simulink model "RoboSoccerSim"  (R2022b)
settings: Solver=ode4  StartTime=0.0  StopTime=inf  FixedStep=0.01  RelTol=1e-3
libraries: dspindex x20
(part 1 of 2)
settings Model: Creator=Wikian  LastModifiedBy=Sahil Gaurkar
settings ModelReferenceCC: EnableRefExpFcnMdlSchedulingChecks=on

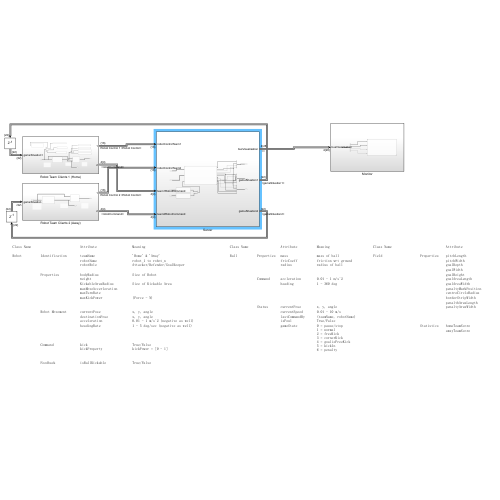
[thumbnail: Simulink's stored preview of the top-level diagram]
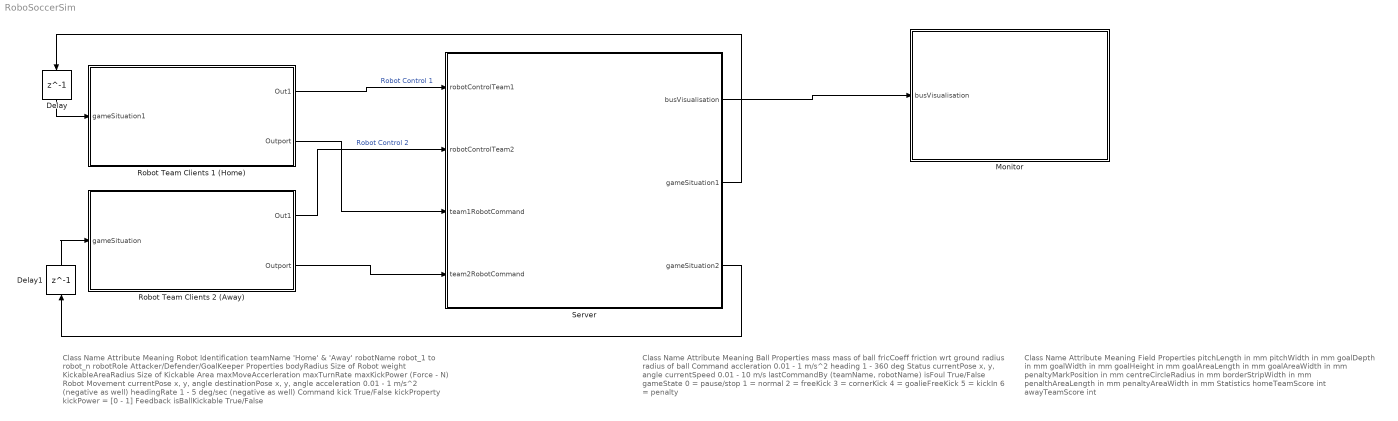
== system RoboSoccerSim ==
  note: Class Name
      |
      | Attribute
      | Meaning
      |
      | Field
      | Properties
      | pitchLength
      | in mm
      |
      | pitchWidth
      | in mm
      |
      | goalDepth
      | in mm
      |
      | goalWidth
      | in mm
      |
      | goalHeight
      | in mm
      |
      | goalAreaLength
      | in mm
      |
      | goalAreaWidth
      | in mm
      |
      | penaltyMarkPosition
      | in mm
      |
      | centreCircleRadius
      | in mm
      |
      | borderStripWidth
      | in mm
      |
      | penalthAreaLength
      | in mm
      |
      | penaltyAreaWidth
      | in mm
      |
      | Statistics
      | homeTeamScore
      | int
      |
      | awayTeamScore
      | int
  note: Class Name
      |
      | Attribute
      | Meaning
      |
      | Ball
      | Properties
      | mass
      | mass of ball
      |
      | fricCoeff
      | friction wrt ground
      |
      | radius
      | radius of ball
      |
      | Command
      | accleration
      | 0.01 - 1 m/s^2
      |
      | heading
      | 1 - 360 deg
      |
      | Status
      | currentPose
      | x, y, angle
      |
      | currentSpeed
      | 0.01 - 10 m/s
      |
      | lastCommandBy
      | (teamName, robotName)
      |
      | isFoul
      | True/False
      |
      | gameState
      | 0 = pause/stop
      | 1 = normal
      | 2 = freeKick
      | 3 = cornerKick
      | 4 = goalieFreeKick
      | 5 = kickIn
      | 6 = penalty
  note: Class Name
      |
      | Attribute
      | Meaning
      |
      | Robot
      | Identification
      | teamName
      | 'Home' & 'Away'
      |
      | robotName
      | robot_1 to robot_n
      |
      | robotRole
      | Attacker/Defender/GoalKeeper
      |
      | Properties
      | bodyRadius
      | Size of Robot
      |
      | weight
      |
      | KickableAreaRadius
      | Size of Kickable Area
      |
      | maxMoveAccerleration
      |
      | maxTurnRate
      |
      | maxKickPower
      | (Force - N)
      |
      | Robot Movement
      | currentPose
      | x, y, angle
      |
      | destinationPose
      | x, y, angle
      |
      | acceleration
      | 0.01 - 1 m/s^2 (negative as well)
      |
      | headingRate
      | 1 - 5 deg/sec (negative as well)
      |
      | Command
      | kick
      | True/False
      |
      | kickProperty
      | kickPower = [0 - 1]
      |
      | Feedback
      | isBallKickable
      | True/False
  Delay : Delay  DelayLength=1
  Delay1 : Delay  DelayLength=1
  Monitor : Subsystem
  Robot Team Clients 1 (Home) : Subsystem
  Robot Team Clients 2 (Away) : Subsystem
  Server : Subsystem
  wires:
  Robot Team Clients 1 (Home)/1(Out1) -> Server/1(robotControlTeam1)  "Robot Control 1"
  Robot Team Clients 2 (Away)/1(Out1) -> Server/2(robotControlTeam2)  "Robot Control 2"
  Server/1(busVisualisation) -> Monitor/1(busVisualisation)
  Server/3(gameSituation2) -> Delay1/1
  Server/2(gameSituation1) -> Delay/1
  Delay/1 -> Robot Team Clients 1 (Home)/1(gameSituation1)
  Delay1/1 -> Robot Team Clients 2 (Away)/1(gameSituation)
  Robot Team Clients 1 (Home)/2(Outport) -> Server/3(team1RobotCommand)
  Robot Team Clients 2 (Away)/2(Outport) -> Server/4(team2RobotCommand)

== system RoboSoccerSim/Monitor ==
  busVisualisation : Inport
  Bus Selector : BusSelector  OutputSignals=robot coordinates and heading,ballCurrentPose,home team score,away team score
  Subsystem Reference : Subsystem  ReferencedSubsystem=Monitor_Subsystem
  wires:
  busVisualisation/1 -> Bus Selector/1
  Bus Selector/1 -> Subsystem Reference/1  "<robot coordinates and heading>"
  Bus Selector/2 -> Subsystem Reference/2  "<ballCurrentPose>"
  Bus Selector/3 -> Subsystem Reference/3  "<home team score>"
  Bus Selector/4 -> Subsystem Reference/4  "<away team score>"

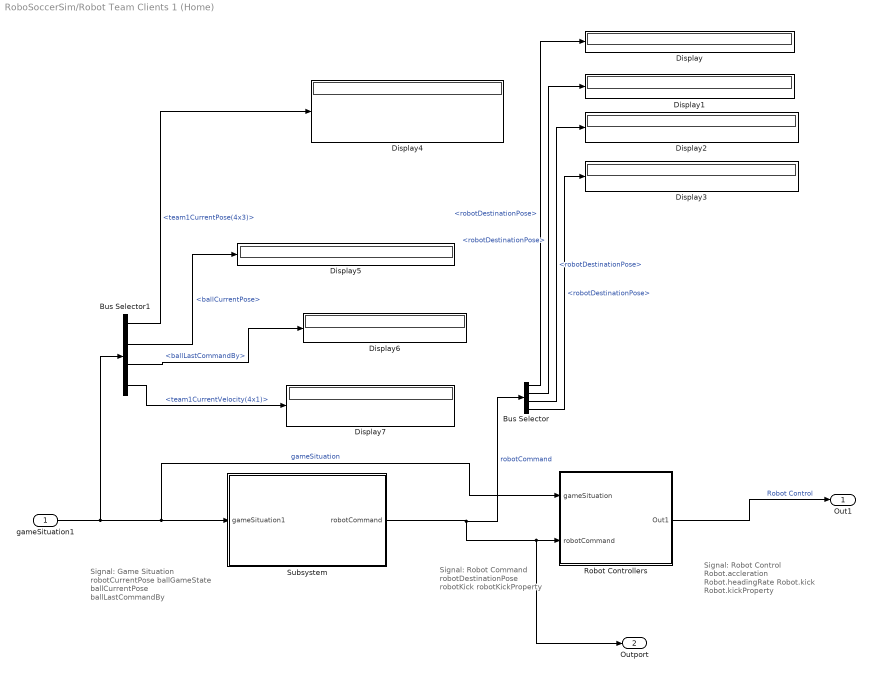
== system RoboSoccerSim/Robot Team Clients 1 (Home) ==
  note: Signal: Robot Control
      |
      | 	Robot.accleration
      | 	Robot.headingRate
      | 	Robot.kick
      | 	Robot.kickProperty
  note: Signal: Robot Command
      |
      | 	robotDestinationPose
      | 	robotKick
      | 	robotKickProperty
  note: Signal: Game Situation
      | 	robotCurrentPose
      | 	ballGameState
      | 	ballCurrentPose
      | 	ballLastCommandBy
  gameSituation1 : Inport  OutDataTypeStr=Bus: gameSituation
  Bus Selector : BusSelector  OutputSignals=robot1.robotDestinationPose,robot2.robotDestinationPose,robot3.robotDestinationPose,robot4.robotDestinationPose
  Bus Selector1 : BusSelector  OutputSignals=team1CurrentPose(4x3),ballCurrentPose,ballLastCommandBy,team1CurrentVelocity(4x1)
  Display{,1..7} (8 alike) : Display
  Robot Controllers : Subsystem
  Subsystem : Subsystem
  Out1 : Outport
  Outport : Outport  Port=2
  wires:
  gameSituation1/1 -> Bus Selector1/1, Subsystem/1(gameSituation1), Robot Controllers/1(gameSituation)  "gameSituation"
  Subsystem/1(robotCommand) -> Bus Selector/1, Outport/1, Robot Controllers/2(robotCommand)  "robotCommand"
  Robot Controllers/1(Out1) -> Out1/1  "Robot Control"
  Bus Selector/1 -> Display/1  "<robotDestinationPose>"
  Bus Selector/2 -> Display1/1  "<robotDestinationPose>"
  Bus Selector/3 -> Display2/1  "<robotDestinationPose>"
  Bus Selector/4 -> Display3/1  "<robotDestinationPose>"
  Bus Selector1/1 -> Display4/1  "<team1CurrentPose(4x3)>"
  Bus Selector1/2 -> Display5/1  "<ballCurrentPose>"
  Bus Selector1/3 -> Display6/1  "<ballLastCommandBy>"
  Bus Selector1/4 -> Display7/1  "<team1CurrentVelocity(4x1)>"

== system RoboSoccerSim/Robot Team Clients 2 (Away) ==
  note: Signal: Robot Control
      |
      | 	Robot.accleration
      | 	Robot.headingRate
      | 	Robot.kick
      | 	Robot.kickProperty
  note: Signal: Robot Command
      |
      | 	robotDestinationPose
      | 	robotKick
      | 	robotKickProperty
  note: Signal: Game Situation
      | 	robotCurrentPose
      | 	ballGameState
      | 	ballCurrentPose
      | 	ballLastCommandBy
  gameSituation : Inport  OutDataTypeStr=Bus:gameSituation
  Robot Controllers : Subsystem
  Subsystem : Subsystem
  Out1 : Outport
  Outport : Outport  Port=2
  wires:
  gameSituation/1 -> Subsystem/1(gameSituation1), Robot Controllers/1(gameSituation)  "gameSituation"
  Subsystem/1(robotCommand) -> Outport/1, Robot Controllers/2(robotCommand)  "robotCommand"
  Robot Controllers/1(Out1) -> Out1/1  "Robot Control"

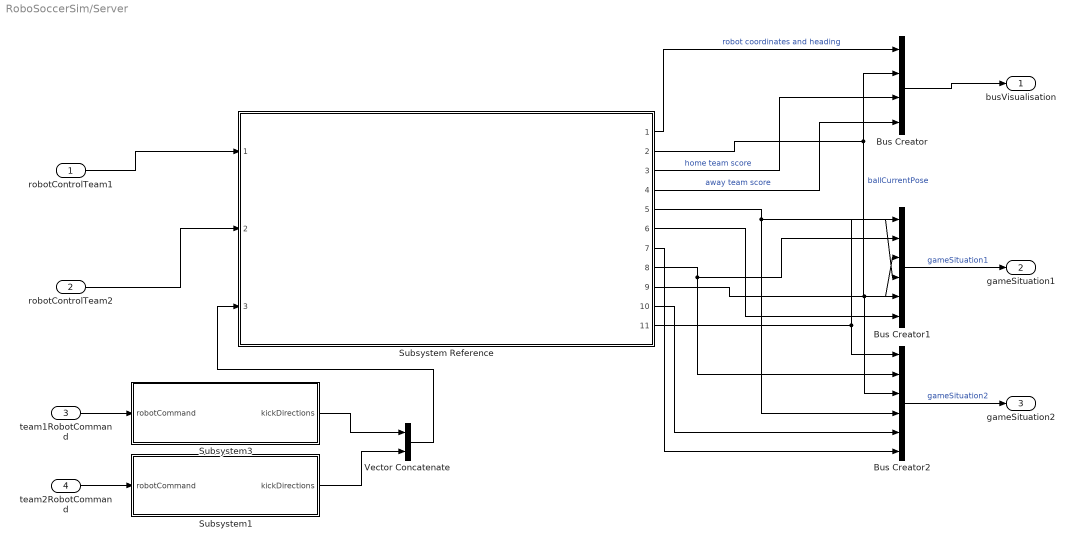
== system RoboSoccerSim/Server ==
  robotControlTeam1 : Inport
  robotControlTeam2 : Inport  Port=2
  team1RobotCommand : Inport  Port=3
  team2RobotCommand : Inport  Port=4
  Bus Creator : BusCreator  Inputs=4
  Bus Creator1 : BusCreator  Inputs=6  OutDataTypeStr=Bus: gameSituation
  Bus Creator2 : BusCreator  Inputs=6  OutDataTypeStr=Bus: gameSituation
  Subsystem Reference : Subsystem  ReferencedSubsystem=Server_sub
  Subsystem1 : Subsystem
  Subsystem3 : Subsystem
  Vector Concatenate : Concatenate
  busVisualisation : Outport
  gameSituation1 : Outport  Port=2
  gameSituation2 : Outport  Port=3
  wires:
  robotControlTeam2/1 -> Subsystem Reference/2
  robotControlTeam1/1 -> Subsystem Reference/1
  Subsystem Reference/1 -> Bus Creator/1  "robot coordinates and heading"
  Subsystem Reference/2 -> Bus Creator/2, Bus Creator2/3, Bus Creator1/3  "ballCurrentPose"
  Subsystem Reference/3 -> Bus Creator/3  "home team score"
  Subsystem Reference/4 -> Bus Creator/4  "away team score"
  Subsystem Reference/5 -> Bus Creator2/4, Bus Creator1/4
  Bus Creator/1 -> busVisualisation/1
  Subsystem Reference/6 -> Bus Creator1/6
  Subsystem Reference/8 -> Bus Creator2/2, Bus Creator1/2
  Subsystem Reference/9 -> Bus Creator1/5
  Subsystem Reference/11 -> Bus Creator2/1, Bus Creator1/1
  Bus Creator1/1 -> gameSituation1/1  "gameSituation1"
  Subsystem Reference/7 -> Bus Creator2/6
  Subsystem Reference/10 -> Bus Creator2/5
  Bus Creator2/1 -> gameSituation2/1  "gameSituation2"
  Vector Concatenate/1 -> Subsystem Reference/3
  team2RobotCommand/1 -> Subsystem1/1(robotCommand)
  Subsystem1/1(kickDirections) -> Vector Concatenate/2
  team1RobotCommand/1 -> Subsystem3/1(robotCommand)
  Subsystem3/1(kickDirections) -> Vector Concatenate/1

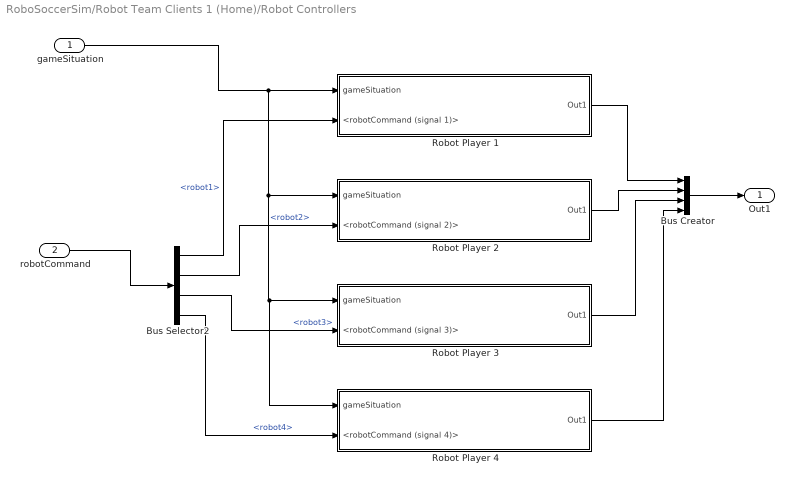
== system RoboSoccerSim/Robot Team Clients 1 (Home)/Robot Controllers ==
  gameSituation : Inport
  robotCommand : Inport  Port=2
  Bus Creator : BusCreator  Inputs=4
  Bus Selector2 : BusSelector  OutputSignals=robot1,robot2,robot3,robot4
  Robot Player 1 : Subsystem
  Robot Player 2 : Subsystem
  Robot Player 3 : Subsystem
  Robot Player 4 : Subsystem
  Out1 : Outport
  wires:
  Robot Player 1/1(Out1) -> Bus Creator/1
  Bus Creator/1 -> Out1/1
  robotCommand/1 -> Bus Selector2/1
  Bus Selector2/1 -> Robot Player 1/2(<robotCommand (signal 1)>)  "<robot1>"
  gameSituation/1 -> Robot Player 4/1(gameSituation), Robot Player 3/1(gameSituation), Robot Player 2/1(gameSituation), Robot Player 1/1(gameSituation)
  Bus Selector2/2 -> Robot Player 2/2(<robotCommand (signal 2)>)  "<robot2>"
  Bus Selector2/3 -> Robot Player 3/2(<robotCommand (signal 3)>)  "<robot3>"
  Robot Player 2/1(Out1) -> Bus Creator/2
  Robot Player 3/1(Out1) -> Bus Creator/3
  Robot Player 4/1(Out1) -> Bus Creator/4
  Bus Selector2/4 -> Robot Player 4/2(<robotCommand (signal 4)>)  "<robot4>"

== system RoboSoccerSim/Robot Team Clients 1 (Home)/Subsystem ==
  gameSituation1 : Inport  OutDataTypeStr=Bus: gameSituation
  Bus Creator : BusCreator  Inputs=4
  Bus Selector : BusSelector  OutputSignals=robotDestinationPose
  Display : Display
  Home Player Strategy 1 : Stateflow chart  TreatAsAtomicUnit=on
  Home Player Strategy 2 : Stateflow chart  TreatAsAtomicUnit=on
  Home Player Strategy 3 : Stateflow chart  TreatAsAtomicUnit=on
  Home Player Strategy 4 : Stateflow chart  TreatAsAtomicUnit=on
  robotCommand : Outport
  wires:
  Home Player Strategy 3/1(robotCommand) -> Bus Creator/3  "robot3"
  gameSituation1/1 -> Home Player Strategy 2/1(gameSituation), Home Player Strategy 1/1(gameSituation), Home Player Strategy 4/1(gameSituation), Home Player Strategy 3/1(gameSituation)  "gameSituation1"
  Home Player Strategy 2/1(robotCommand) -> Bus Creator/2  "robot2"
  Bus Selector/1 -> Display/1  "<robotDestinationPose>"
  Home Player Strategy 4/1(robotCommand) -> Bus Creator/4  "robot4"
  Home Player Strategy 1/1(robotCommand) -> Bus Selector/1, Bus Creator/1  "robot1"
  Bus Creator/1 -> robotCommand/1

== system RoboSoccerSim/Robot Team Clients 2 (Away)/Robot Controllers ==
  gameSituation : Inport
  robotCommand : Inport  Port=2
  Bus Creator : BusCreator  Inputs=4
  Bus Selector2 : BusSelector  OutputSignals=robot1,robot2,robot3,robot4
  Robot Player 1 : Subsystem
  Robot Player 2 : Subsystem
  Robot Player 3 : Subsystem
  Robot Player 4 : Subsystem
  Out1 : Outport
  wires:
  Robot Player 1/1(Out1) -> Bus Creator/1
  Bus Creator/1 -> Out1/1
  robotCommand/1 -> Bus Selector2/1
  Bus Selector2/1 -> Robot Player 1/2(<robotCommand (signal 1)>)  "<robot1>"
  gameSituation/1 -> Robot Player 4/1(gameSituation), Robot Player 3/1(gameSituation), Robot Player 2/1(gameSituation), Robot Player 1/1(gameSituation)
  Bus Selector2/2 -> Robot Player 2/2(<robotCommand (signal 2)>)  "<robot2>"
  Bus Selector2/3 -> Robot Player 3/2(<robotCommand (signal 3)>)  "<robot3>"
  Robot Player 2/1(Out1) -> Bus Creator/2
  Robot Player 3/1(Out1) -> Bus Creator/3
  Robot Player 4/1(Out1) -> Bus Creator/4
  Bus Selector2/4 -> Robot Player 4/2(<robotCommand (signal 4)>)  "<robot4>"

== system RoboSoccerSim/Robot Team Clients 2 (Away)/Subsystem ==
  gameSituation1 : Inport  OutDataTypeStr=Bus: gameSituation
  Away Player Strategy 1 : Stateflow chart  TreatAsAtomicUnit=on
  Away Player Strategy 2 : Stateflow chart  TreatAsAtomicUnit=on
  Away Player Strategy 3 : Stateflow chart  TreatAsAtomicUnit=on
  Away Player Strategy 4 : Stateflow chart  TreatAsAtomicUnit=on
  Bus Creator : BusCreator  Inputs=4
  Bus Selector : BusSelector  OutputSignals=robotDestinationPose
  Display : Display
  robotCommand : Outport
  wires:
  Away Player Strategy 3/1(robotCommand) -> Bus Creator/3  "robot3"
  gameSituation1/1 -> Away Player Strategy 2/1(gameSituation), Away Player Strategy 1/1(gameSituation), Away Player Strategy 4/1(gameSituation), Away Player Strategy 3/1(gameSituation)  "gameSituation1"
  Away Player Strategy 2/1(robotCommand) -> Bus Creator/2  "robot2"
  Bus Selector/1 -> Display/1  "<robotDestinationPose>"
  Away Player Strategy 4/1(robotCommand) -> Bus Creator/4  "robot4"
  Away Player Strategy 1/1(robotCommand) -> Bus Creator/1, Bus Selector/1  "robot1"
  Bus Creator/1 -> robotCommand/1

== system RoboSoccerSim/Server/Subsystem1 ==
  note: Signal: Robot Control
      |
      | 	Robot.accleration
      | 	Robot.headingRate
      | 	Robot.kick
      | 	Robot.kickProperty
  robotCommand : Inport
  Bus Selector2 : BusSelector  OutputSignals=robot1.robotDestinationPose,robot2.robotDestinationPose,robot3.robotDestinationPose,robot4.robotDestinationPose
  MATLAB Function : MATLAB Function  TreatAsAtomicUnit=on
  MATLAB Function1 : MATLAB Function  TreatAsAtomicUnit=on
  MATLAB Function2 : MATLAB Function  TreatAsAtomicUnit=on
  MATLAB Function3 : MATLAB Function  TreatAsAtomicUnit=on
  Vector Concatenate : Concatenate  NumInputs=4
  kickDirections : Outport
  wires:
  MATLAB Function/1(kickDirection) -> Vector Concatenate/1
  Vector Concatenate/1 -> kickDirections/1
  MATLAB Function1/1(kickDirection) -> Vector Concatenate/2
  robotCommand/1 -> Bus Selector2/1
  Bus Selector2/4 -> MATLAB Function3/1(destinationPose)  "<robotDestinationPose>"
  Bus Selector2/1 -> MATLAB Function/1(destinationPose)  "<robotDestinationPose>"
  MATLAB Function2/1(kickDirection) -> Vector Concatenate/3
  Bus Selector2/2 -> MATLAB Function1/1(destinationPose)  "<robotDestinationPose>"
  Bus Selector2/3 -> MATLAB Function2/1(destinationPose)  "<robotDestinationPose>"
  MATLAB Function3/1(kickDirection) -> Vector Concatenate/4

== system RoboSoccerSim/Server/Subsystem3 ==
  note: Signal: Robot Control
      |
      | 	Robot.accleration
      | 	Robot.headingRate
      | 	Robot.kick
      | 	Robot.kickProperty
  robotCommand : Inport
  Bus Selector2 : BusSelector  OutputSignals=robot1.robotDestinationPose,robot2.robotDestinationPose,robot3.robotDestinationPose,robot4.robotDestinationPose
  MATLAB Function : MATLAB Function  TreatAsAtomicUnit=on
  MATLAB Function1 : MATLAB Function  TreatAsAtomicUnit=on
  MATLAB Function2 : MATLAB Function  TreatAsAtomicUnit=on
  MATLAB Function3 : MATLAB Function  TreatAsAtomicUnit=on
  Vector Concatenate : Concatenate  NumInputs=4
  kickDirections : Outport
  wires:
  MATLAB Function/1(kickDirection) -> Vector Concatenate/1
  Vector Concatenate/1 -> kickDirections/1
  MATLAB Function1/1(kickDirection) -> Vector Concatenate/2
  robotCommand/1 -> Bus Selector2/1
  Bus Selector2/4 -> MATLAB Function3/1(destinationPose)  "<robotDestinationPose>"
  Bus Selector2/1 -> MATLAB Function/1(destinationPose)  "<robotDestinationPose>"
  MATLAB Function2/1(kickDirection) -> Vector Concatenate/3
  Bus Selector2/2 -> MATLAB Function1/1(destinationPose)  "<robotDestinationPose>"
  Bus Selector2/3 -> MATLAB Function2/1(destinationPose)  "<robotDestinationPose>"
  MATLAB Function3/1(kickDirection) -> Vector Concatenate/4

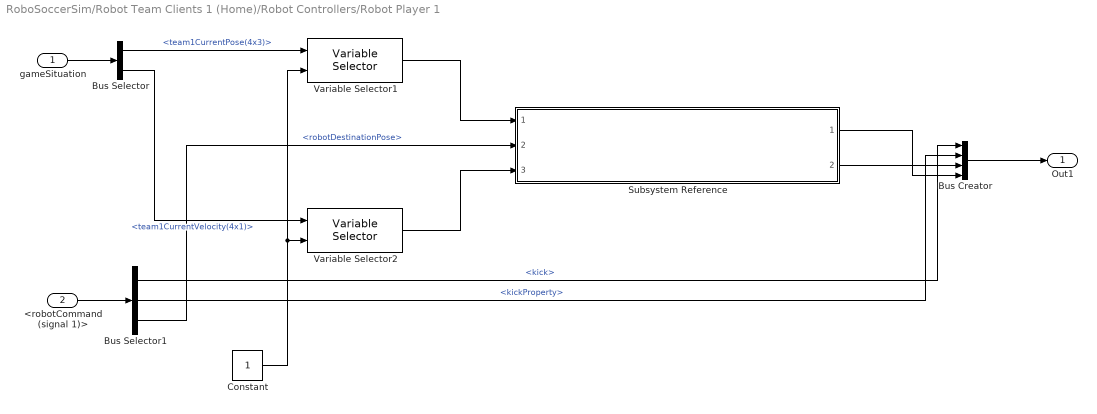
== system RoboSoccerSim/Robot Team Clients 1 (Home)/Robot Controllers/Robot Player 1 ==
  gameSituation : Inport
  <robotCommand (signal 1)> : Inport  Port=2
  Bus Creator : BusCreator  Inputs=4  OutDataTypeStr=Bus: robotControl
  Bus Selector : BusSelector  OutputSignals=team1CurrentPose(4x3),team1CurrentVelocity(4x1)
  Bus Selector1 : BusSelector  OutputSignals=kick,kickProperty,robotDestinationPose
  Constant : Constant
  Subsystem Reference : Subsystem  ReferencedSubsystem=Controller_Subsystem
  Variable Selector1 : dspindex/Variable Selector  NumInputs=1  rowsOrCols=Rows  IdxMode=Variable  Elements=[1 3]  ZerOneIdxMode=One-based  errmode=Clip Index  FillMode=on  FillValues=0
      settings: LibrarySourceBlock=|
      | dsphdlsupportsigmgmt/Variable
      | Selector
  Variable Selector2 : dspindex/Variable Selector  NumInputs=1  rowsOrCols=Rows  IdxMode=Variable  Elements=[1 3]  ZerOneIdxMode=One-based  errmode=Clip Index  FillMode=on  FillValues=0
      settings: LibrarySourceBlock=|
      | dsphdlsupportsigmgmt/Variable
      | Selector
  Out1 : Outport
  wires:
  Bus Selector1/3 -> Subsystem Reference/2  "<robotDestinationPose>"
  Constant/1 -> Variable Selector2/2, Variable Selector1/2
  Variable Selector1/1 -> Subsystem Reference/1
  Variable Selector2/1 -> Subsystem Reference/3
  gameSituation/1 -> Bus Selector/1
  Bus Selector/1 -> Variable Selector1/1  "<team1CurrentPose(4x3)>"
  Bus Selector/2 -> Variable Selector2/1  "<team1CurrentVelocity(4x1)>"
  <robotCommand (signal 1)>/1 -> Bus Selector1/1
  Bus Selector1/1 -> Bus Creator/1  "<kick>"
  Bus Selector1/2 -> Bus Creator/2  "<kickProperty>"
  Subsystem Reference/1 -> Bus Creator/4
  Subsystem Reference/2 -> Bus Creator/3
  Bus Creator/1 -> Out1/1

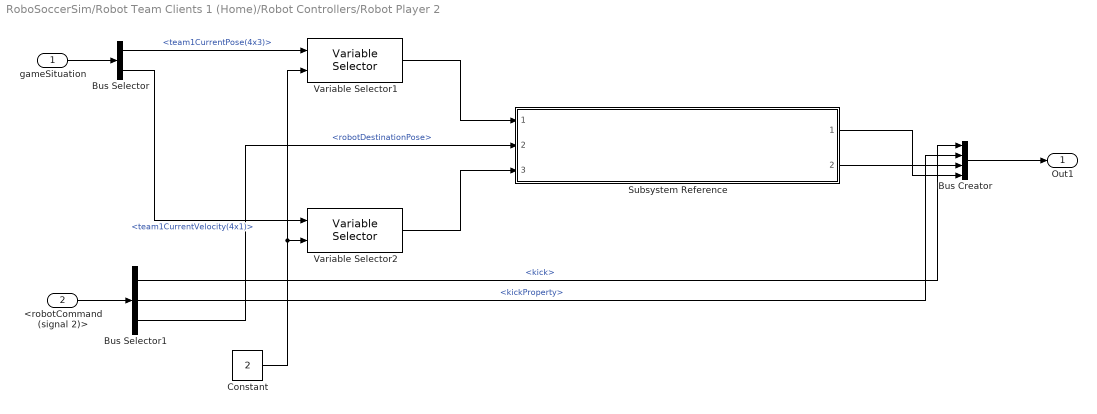
== system RoboSoccerSim/Robot Team Clients 1 (Home)/Robot Controllers/Robot Player 2 ==
  gameSituation : Inport
  <robotCommand (signal 2)> : Inport  Port=2
  Bus Creator : BusCreator  Inputs=4  OutDataTypeStr=Bus: robotControl
  Bus Selector : BusSelector  OutputSignals=team1CurrentPose(4x3),team1CurrentVelocity(4x1)
  Bus Selector1 : BusSelector  OutputSignals=kick,kickProperty,robotDestinationPose
  Constant : Constant  Value=2
  Subsystem Reference : Subsystem  ReferencedSubsystem=Controller_Subsystem
  Variable Selector1 : dspindex/Variable Selector  NumInputs=1  rowsOrCols=Rows  IdxMode=Variable  Elements=[1 3]  ZerOneIdxMode=One-based  errmode=Clip Index  FillMode=on  FillValues=0
      settings: LibrarySourceBlock=|
      | dsphdlsupportsigmgmt/Variable
      | Selector
  Variable Selector2 : dspindex/Variable Selector  NumInputs=1  rowsOrCols=Rows  IdxMode=Variable  Elements=[1 3]  ZerOneIdxMode=One-based  errmode=Clip Index  FillMode=on  FillValues=0
      settings: LibrarySourceBlock=|
      | dsphdlsupportsigmgmt/Variable
      | Selector
  Out1 : Outport
  wires:
  Constant/1 -> Variable Selector2/2, Variable Selector1/2
  Variable Selector1/1 -> Subsystem Reference/1
  Variable Selector2/1 -> Subsystem Reference/3
  gameSituation/1 -> Bus Selector/1
  Bus Selector/1 -> Variable Selector1/1  "<team1CurrentPose(4x3)>"
  Bus Selector/2 -> Variable Selector2/1  "<team1CurrentVelocity(4x1)>"
  <robotCommand (signal 2)>/1 -> Bus Selector1/1
  Bus Selector1/1 -> Bus Creator/1  "<kick>"
  Bus Selector1/2 -> Bus Creator/2  "<kickProperty>"
  Subsystem Reference/1 -> Bus Creator/4
  Subsystem Reference/2 -> Bus Creator/3
  Bus Creator/1 -> Out1/1
  Bus Selector1/3 -> Subsystem Reference/2  "<robotDestinationPose>"

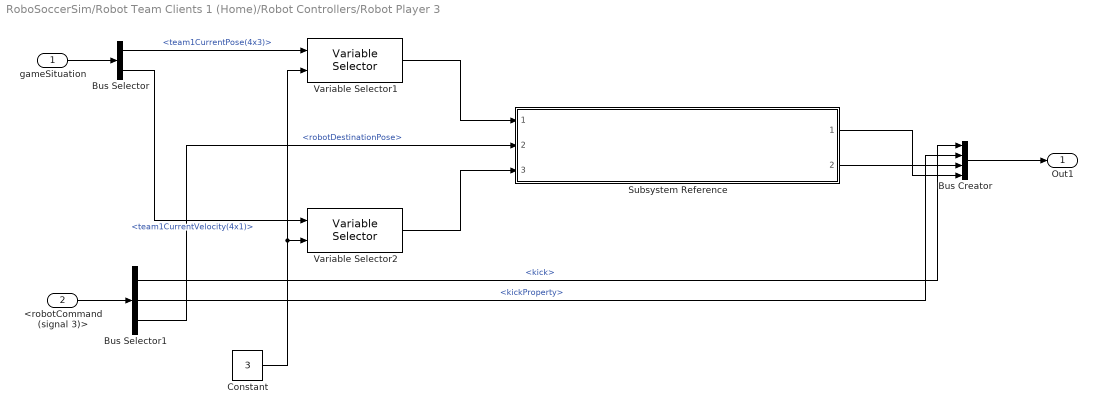
== system RoboSoccerSim/Robot Team Clients 1 (Home)/Robot Controllers/Robot Player 3 ==
  gameSituation : Inport
  <robotCommand (signal 3)> : Inport  Port=2
  Bus Creator : BusCreator  Inputs=4  OutDataTypeStr=Bus: robotControl
  Bus Selector : BusSelector  OutputSignals=team1CurrentPose(4x3),team1CurrentVelocity(4x1)
  Bus Selector1 : BusSelector  OutputSignals=kick,kickProperty,robotDestinationPose
  Constant : Constant  Value=3
  Subsystem Reference : Subsystem  ReferencedSubsystem=Controller_Subsystem
  Variable Selector1 : dspindex/Variable Selector  NumInputs=1  rowsOrCols=Rows  IdxMode=Variable  Elements=[1 3]  ZerOneIdxMode=One-based  errmode=Clip Index  FillMode=on  FillValues=0
      settings: LibrarySourceBlock=|
      | dsphdlsupportsigmgmt/Variable
      | Selector
  Variable Selector2 : dspindex/Variable Selector  NumInputs=1  rowsOrCols=Rows  IdxMode=Variable  Elements=[1 3]  ZerOneIdxMode=One-based  errmode=Clip Index  FillMode=on  FillValues=0
      settings: LibrarySourceBlock=|
      | dsphdlsupportsigmgmt/Variable
      | Selector
  Out1 : Outport
  wires:
  Bus Selector1/3 -> Subsystem Reference/2  "<robotDestinationPose>"
  Constant/1 -> Variable Selector2/2, Variable Selector1/2
  Variable Selector1/1 -> Subsystem Reference/1
  Variable Selector2/1 -> Subsystem Reference/3
  gameSituation/1 -> Bus Selector/1
  Bus Selector/1 -> Variable Selector1/1  "<team1CurrentPose(4x3)>"
  Bus Selector/2 -> Variable Selector2/1  "<team1CurrentVelocity(4x1)>"
  <robotCommand (signal 3)>/1 -> Bus Selector1/1
  Bus Selector1/1 -> Bus Creator/1  "<kick>"
  Bus Selector1/2 -> Bus Creator/2  "<kickProperty>"
  Subsystem Reference/1 -> Bus Creator/4
  Subsystem Reference/2 -> Bus Creator/3
  Bus Creator/1 -> Out1/1

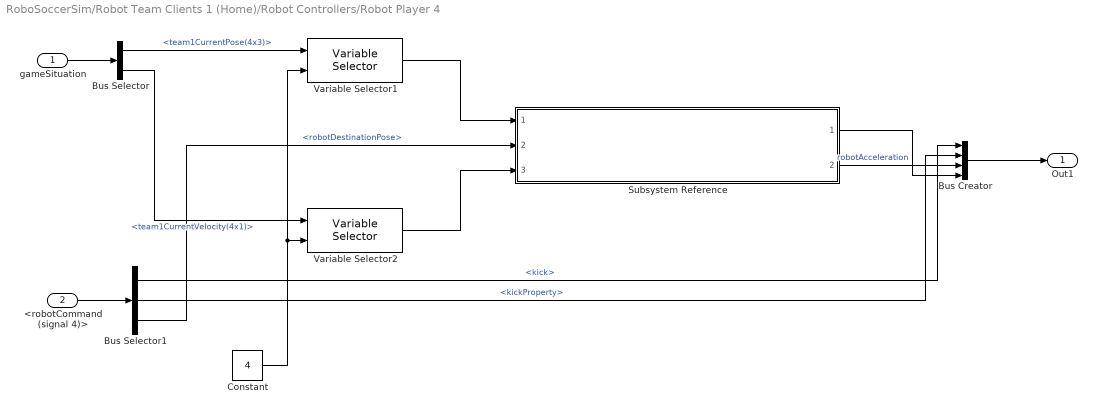
== system RoboSoccerSim/Robot Team Clients 1 (Home)/Robot Controllers/Robot Player 4 ==
  gameSituation : Inport
  <robotCommand (signal 4)> : Inport  Port=2
  Bus Creator : BusCreator  Inputs=4  OutDataTypeStr=Bus: robotControl
  Bus Selector : BusSelector  OutputSignals=team1CurrentPose(4x3),team1CurrentVelocity(4x1)
  Bus Selector1 : BusSelector  OutputSignals=kick,kickProperty,robotDestinationPose
  Constant : Constant  Value=4
  Subsystem Reference : Subsystem  ReferencedSubsystem=Controller_Subsystem
  Variable Selector1 : dspindex/Variable Selector  NumInputs=1  rowsOrCols=Rows  IdxMode=Variable  Elements=[1 3]  ZerOneIdxMode=One-based  errmode=Clip Index  FillMode=on  FillValues=0
      settings: LibrarySourceBlock=|
      | dsphdlsupportsigmgmt/Variable
      | Selector
  Variable Selector2 : dspindex/Variable Selector  NumInputs=1  rowsOrCols=Rows  IdxMode=Variable  Elements=[1 3]  ZerOneIdxMode=One-based  errmode=Clip Index  FillMode=on  FillValues=0
      settings: LibrarySourceBlock=|
      | dsphdlsupportsigmgmt/Variable
      | Selector
  Out1 : Outport
  wires:
  Bus Selector1/3 -> Subsystem Reference/2  "<robotDestinationPose>"
  Constant/1 -> Variable Selector2/2, Variable Selector1/2
  Variable Selector1/1 -> Subsystem Reference/1
  Variable Selector2/1 -> Subsystem Reference/3
  gameSituation/1 -> Bus Selector/1
  Bus Selector/1 -> Variable Selector1/1  "<team1CurrentPose(4x3)>"
  Bus Selector/2 -> Variable Selector2/1  "<team1CurrentVelocity(4x1)>"
  <robotCommand (signal 4)>/1 -> Bus Selector1/1
  Bus Selector1/1 -> Bus Creator/1  "<kick>"
  Bus Selector1/2 -> Bus Creator/2  "<kickProperty>"
  Subsystem Reference/1 -> Bus Creator/4
  Subsystem Reference/2 -> Bus Creator/3  "robotAcceleration"
  Bus Creator/1 -> Out1/1

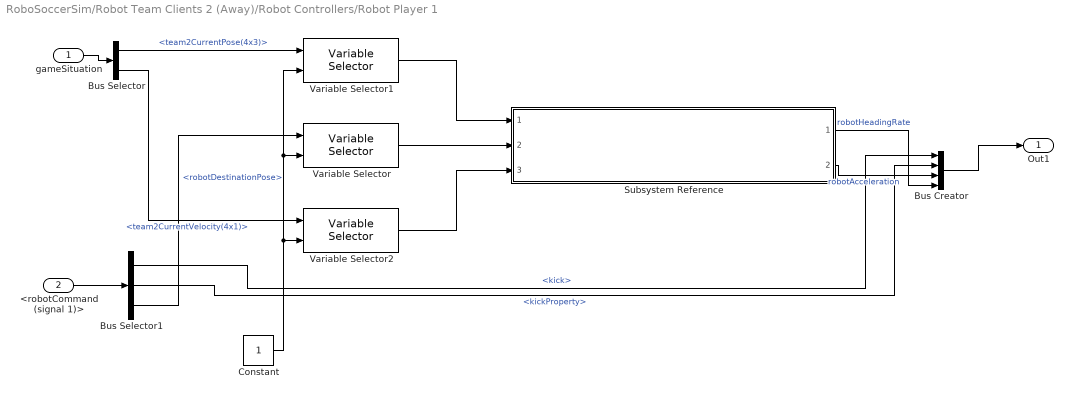
== system RoboSoccerSim/Robot Team Clients 2 (Away)/Robot Controllers/Robot Player 1 ==
  gameSituation : Inport
  <robotCommand (signal 1)> : Inport  Port=2
  Bus Creator : BusCreator  Inputs=4  OutDataTypeStr=Bus: robotControl
  Bus Selector : BusSelector  OutputSignals=team2CurrentPose(4x3),team2CurrentVelocity(4x1)
  Bus Selector1 : BusSelector  OutputSignals=kick,kickProperty,robotDestinationPose
  Constant : Constant
  Subsystem Reference : Subsystem  ReferencedSubsystem=Controller_Subsystem
  Variable Selector : dspindex/Variable Selector  NumInputs=1  rowsOrCols=Rows  IdxMode=Variable  Elements=[1 3]  ZerOneIdxMode=One-based  errmode=Clip Index  FillMode=on  FillValues=0
      settings: LibrarySourceBlock=|
      | dsphdlsupportsigmgmt/Variable
      | Selector
  Variable Selector1 : dspindex/Variable Selector  NumInputs=1  rowsOrCols=Rows  IdxMode=Variable  Elements=[1 3]  ZerOneIdxMode=One-based  errmode=Clip Index  FillMode=on  FillValues=0
      settings: LibrarySourceBlock=|
      | dsphdlsupportsigmgmt/Variable
      | Selector
  Variable Selector2 : dspindex/Variable Selector  NumInputs=1  rowsOrCols=Rows  IdxMode=Variable  Elements=[1 3]  ZerOneIdxMode=One-based  errmode=Clip Index  FillMode=on  FillValues=0
      settings: LibrarySourceBlock=|
      | dsphdlsupportsigmgmt/Variable
      | Selector
  Out1 : Outport
  wires:
  Bus Selector1/3 -> Variable Selector/1  "<robotDestinationPose>"
  Variable Selector/1 -> Subsystem Reference/2
  Constant/1 -> Variable Selector2/2, Variable Selector1/2, Variable Selector/2
  Variable Selector1/1 -> Subsystem Reference/1
  Variable Selector2/1 -> Subsystem Reference/3
  gameSituation/1 -> Bus Selector/1
  Bus Selector/2 -> Variable Selector2/1  "<team2CurrentVelocity(4x1)>"
  <robotCommand (signal 1)>/1 -> Bus Selector1/1
  Bus Selector1/1 -> Bus Creator/1  "<kick>"
  Bus Selector1/2 -> Bus Creator/2  "<kickProperty>"
  Subsystem Reference/1 -> Bus Creator/4  "robotHeadingRate"
  Subsystem Reference/2 -> Bus Creator/3  "robotAcceleration"
  Bus Creator/1 -> Out1/1
  Bus Selector/1 -> Variable Selector1/1  "<team2CurrentPose(4x3)>"

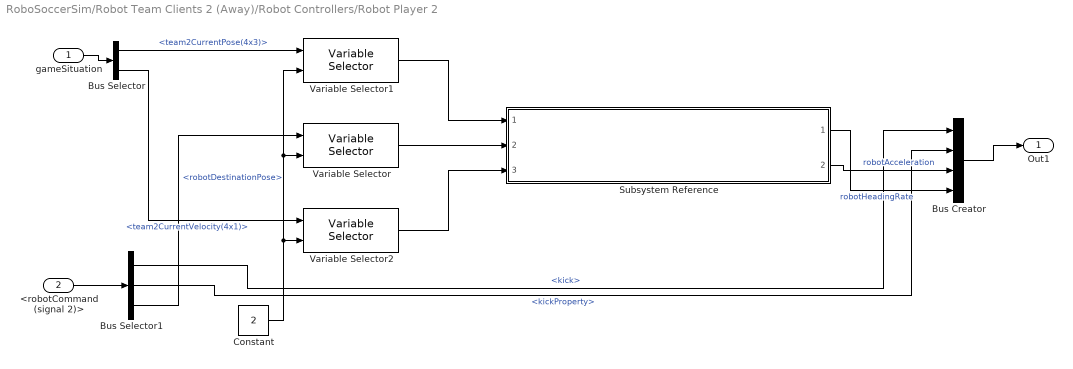
== system RoboSoccerSim/Robot Team Clients 2 (Away)/Robot Controllers/Robot Player 2 ==
  gameSituation : Inport
  <robotCommand (signal 2)> : Inport  Port=2
  Bus Creator : BusCreator  Inputs=4  OutDataTypeStr=Bus: robotControl
  Bus Selector : BusSelector  OutputSignals=team2CurrentPose(4x3),team2CurrentVelocity(4x1)
  Bus Selector1 : BusSelector  OutputSignals=kick,kickProperty,robotDestinationPose
  Constant : Constant  Value=2
  Subsystem Reference : Subsystem  ReferencedSubsystem=Controller_Subsystem
  Variable Selector : dspindex/Variable Selector  NumInputs=1  rowsOrCols=Rows  IdxMode=Variable  Elements=[1 3]  ZerOneIdxMode=One-based  errmode=Clip Index  FillMode=on  FillValues=0
      settings: LibrarySourceBlock=|
      | dsphdlsupportsigmgmt/Variable
      | Selector
  Variable Selector1 : dspindex/Variable Selector  NumInputs=1  rowsOrCols=Rows  IdxMode=Variable  Elements=[1 3]  ZerOneIdxMode=One-based  errmode=Clip Index  FillMode=on  FillValues=0
      settings: LibrarySourceBlock=|
      | dsphdlsupportsigmgmt/Variable
      | Selector
  Variable Selector2 : dspindex/Variable Selector  NumInputs=1  rowsOrCols=Rows  IdxMode=Variable  Elements=[1 3]  ZerOneIdxMode=One-based  errmode=Clip Index  FillMode=on  FillValues=0
      settings: LibrarySourceBlock=|
      | dsphdlsupportsigmgmt/Variable
      | Selector
  Out1 : Outport
  wires:
  Bus Selector1/3 -> Variable Selector/1  "<robotDestinationPose>"
  Variable Selector/1 -> Subsystem Reference/2
  Constant/1 -> Variable Selector2/2, Variable Selector1/2, Variable Selector/2
  Variable Selector1/1 -> Subsystem Reference/1
  Variable Selector2/1 -> Subsystem Reference/3
  gameSituation/1 -> Bus Selector/1
  Bus Selector/2 -> Variable Selector2/1  "<team2CurrentVelocity(4x1)>"
  <robotCommand (signal 2)>/1 -> Bus Selector1/1
  Bus Selector1/1 -> Bus Creator/1  "<kick>"
  Bus Selector1/2 -> Bus Creator/2  "<kickProperty>"
  Subsystem Reference/1 -> Bus Creator/4  "robotHeadingRate"
  Subsystem Reference/2 -> Bus Creator/3  "robotAcceleration"
  Bus Creator/1 -> Out1/1
  Bus Selector/1 -> Variable Selector1/1  "<team2CurrentPose(4x3)>"

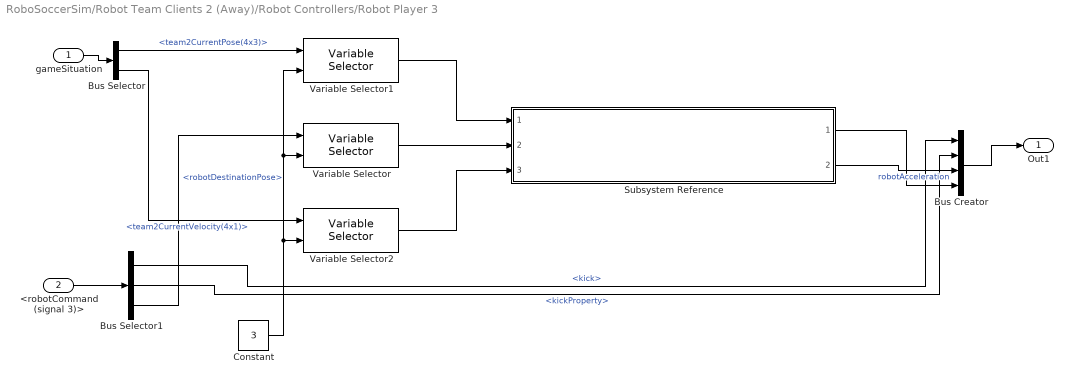
== system RoboSoccerSim/Robot Team Clients 2 (Away)/Robot Controllers/Robot Player 3 ==
  gameSituation : Inport
  <robotCommand (signal 3)> : Inport  Port=2
  Bus Creator : BusCreator  Inputs=4  OutDataTypeStr=Bus: robotControl
  Bus Selector : BusSelector  OutputSignals=team2CurrentPose(4x3),team2CurrentVelocity(4x1)
  Bus Selector1 : BusSelector  OutputSignals=kick,kickProperty,robotDestinationPose
  Constant : Constant  Value=3
  Subsystem Reference : Subsystem  ReferencedSubsystem=Controller_Subsystem
  Variable Selector : dspindex/Variable Selector  NumInputs=1  rowsOrCols=Rows  IdxMode=Variable  Elements=[1 3]  ZerOneIdxMode=One-based  errmode=Clip Index  FillMode=on  FillValues=0
      settings: LibrarySourceBlock=|
      | dsphdlsupportsigmgmt/Variable
      | Selector
  Variable Selector1 : dspindex/Variable Selector  NumInputs=1  rowsOrCols=Rows  IdxMode=Variable  Elements=[1 3]  ZerOneIdxMode=One-based  errmode=Clip Index  FillMode=on  FillValues=0
      settings: LibrarySourceBlock=|
      | dsphdlsupportsigmgmt/Variable
      | Selector
  Variable Selector2 : dspindex/Variable Selector  NumInputs=1  rowsOrCols=Rows  IdxMode=Variable  Elements=[1 3]  ZerOneIdxMode=One-based  errmode=Clip Index  FillMode=on  FillValues=0
      settings: LibrarySourceBlock=|
      | dsphdlsupportsigmgmt/Variable
      | Selector
  Out1 : Outport
  wires:
  Bus Selector1/3 -> Variable Selector/1  "<robotDestinationPose>"
  Variable Selector/1 -> Subsystem Reference/2
  Constant/1 -> Variable Selector2/2, Variable Selector1/2, Variable Selector/2
  Variable Selector1/1 -> Subsystem Reference/1
  Variable Selector2/1 -> Subsystem Reference/3
  gameSituation/1 -> Bus Selector/1
  Bus Selector/2 -> Variable Selector2/1  "<team2CurrentVelocity(4x1)>"
  <robotCommand (signal 3)>/1 -> Bus Selector1/1
  Bus Selector1/1 -> Bus Creator/1  "<kick>"
  Bus Selector1/2 -> Bus Creator/2  "<kickProperty>"
  Subsystem Reference/1 -> Bus Creator/4
  Subsystem Reference/2 -> Bus Creator/3  "robotAcceleration"
  Bus Creator/1 -> Out1/1
  Bus Selector/1 -> Variable Selector1/1  "<team2CurrentPose(4x3)>"

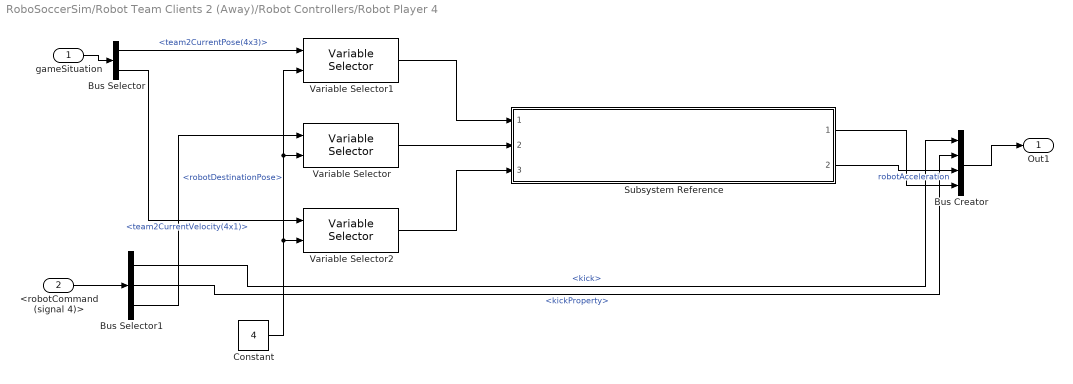
== system RoboSoccerSim/Robot Team Clients 2 (Away)/Robot Controllers/Robot Player 4 ==
  gameSituation : Inport
  <robotCommand (signal 4)> : Inport  Port=2
  Bus Creator : BusCreator  Inputs=4  OutDataTypeStr=Bus: robotControl
  Bus Selector : BusSelector  OutputSignals=team2CurrentPose(4x3),team2CurrentVelocity(4x1)
  Bus Selector1 : BusSelector  OutputSignals=kick,kickProperty,robotDestinationPose
  Constant : Constant  Value=4
  Subsystem Reference : Subsystem  ReferencedSubsystem=Controller_Subsystem
  Variable Selector : dspindex/Variable Selector  NumInputs=1  rowsOrCols=Rows  IdxMode=Variable  Elements=[1 3]  ZerOneIdxMode=One-based  errmode=Clip Index  FillMode=on  FillValues=0
      settings: LibrarySourceBlock=|
      | dsphdlsupportsigmgmt/Variable
      | Selector
  Variable Selector1 : dspindex/Variable Selector  NumInputs=1  rowsOrCols=Rows  IdxMode=Variable  Elements=[1 3]  ZerOneIdxMode=One-based  errmode=Clip Index  FillMode=on  FillValues=0
      settings: LibrarySourceBlock=|
      | dsphdlsupportsigmgmt/Variable
      | Selector
  Variable Selector2 : dspindex/Variable Selector  NumInputs=1  rowsOrCols=Rows  IdxMode=Variable  Elements=[1 3]  ZerOneIdxMode=One-based  errmode=Clip Index  FillMode=on  FillValues=0
      settings: LibrarySourceBlock=|
      | dsphdlsupportsigmgmt/Variable
      | Selector
  Out1 : Outport
  wires:
  Bus Selector1/3 -> Variable Selector/1  "<robotDestinationPose>"
  Variable Selector/1 -> Subsystem Reference/2
  Constant/1 -> Variable Selector2/2, Variable Selector1/2, Variable Selector/2
  Variable Selector1/1 -> Subsystem Reference/1
  Variable Selector2/1 -> Subsystem Reference/3
  gameSituation/1 -> Bus Selector/1
  Bus Selector/2 -> Variable Selector2/1  "<team2CurrentVelocity(4x1)>"
  <robotCommand (signal 4)>/1 -> Bus Selector1/1
  Bus Selector1/1 -> Bus Creator/1  "<kick>"
  Bus Selector1/2 -> Bus Creator/2  "<kickProperty>"
  Subsystem Reference/1 -> Bus Creator/4
  Subsystem Reference/2 -> Bus Creator/3  "robotAcceleration"
  Bus Creator/1 -> Out1/1
  Bus Selector/1 -> Variable Selector1/1  "<team2CurrentPose(4x3)>"

== stateflow chart RoboSoccerSim/Robot Team Clients 2 (Away)/Subsystem/Away Player Strategy 1 ==
  state InitialState
    en,du:
    if gameSituation.kickConfirmation == true
    robotCommand.kick = false;
    end
    id = 1; % Team1(Home) Robot 1
    shootDistThres = 2500;
    kickableAreaRadius = 20;
    homeGoalPose = [5000, 0];
    awayGoalPose = [-5000, 0];
    homeAttackPositions = [[-2500, 0, 180]; [-1500, 2000, 180]; [-1500, -2000, 180]; [2000, 0, 180]];
    homeDefendPositions = [[1000, 0, 180]; [3000, 2000, 180]; [3000, -2000, 180]; [3500, 0, 180]];
  state ROBOT 1 [group]
    (Strategy for robot 1~3)
  state Attack
    en,du:
    %%calculate the distance to the goal
    teamDistToGoal = [0 0 0 0];
    for idx=1:1:4
    teamDistToGoal(idx) = distTo(gameSituation.robotCurrentPose(idx,1:2), awayGoalPose);
    end
    distToGoal1 = distTo(gameSituation.robotCurrentPose(id,1:2), awayGoalPose);
    %calculate the distance to the ball
    teamDistToBall = [0 0 0 0];
    for idx=1:1:4
    teamDistToBall(idx) = distTo(gameSituation.robotCurrentPose(idx,1:2), ...
    gameSituation.ballCurrentPose(1:2));
    end
    distToBall = distTo(gameSituation.robotCurrentPose(id,1:2), ...
    gameSituation.ballCurrentPose(1:2));
  state Defend
    en,du:
    %%calculate the distance to the home goal
    teamDistToOwnGoal = [0 0 0 0];
    for idx=1:1:4
    teamDistToOwnGoal(idx) = distTo(gameSituation.robotCurrentPose(idx,1:2), homeGoalPose);
    end
    distToOwnGoal = distTo(gameSituation.robotCurrentPose(id,1:2), homeGoalPose);
    for idx=1:1:4
    teamDistToBall(idx) = distTo(gameSituation.robotCurrentPose(idx,1:2), ...
    gameSituation.ballCurrentPose(1:2));
    end
    distToBall = distTo(gameSituation.robotCurrentPose(id,1:2), ...
    gameSituation.ballCurrentPose(1:2));
  state Position
    en,du:
    playerAttackPosition = homeAttackPositions(id, :);
    kickPower = 1;
    kickState = false;
    desiredPosition = playerAttackPosition;
    isdone = true;
  state Shoot
    en,du:
    angleBallGoal = atan2d(awayGoalPose(2) - gameSituation.ballCurrentPose(2), ...
    awayGoalPose(1) - gameSituation.ballCurrentPose(1));
    kickPower = 100;
    kickState = true;
    kickDirection = angleBallGoal;
    xPosition= gameSituation.ballCurrentPose(1) + cosd(180 - angleBallGoal) * kickableAreaRadius;
    yPosition = gameSituation.ballCurrentPose(2) + sind(180 - angleBallGoal) * kickableAreaRadius;
    desiredPosition = [xPosition, yPosition, kickDirection];
    isdone = true;
  state Pass
    en,du:
    [minval,minidx] = min(teamDistToGoal)
    angleBallPlayer = atan2d(gameSituation.robotCurrentPose(minidx, 2) - gameSituation.ballCurrentPose(2), ...
    gameSituation.robotCurrentPose(minidx, 1) - gameSituation.ballCurrentPose(1));
    kickPower = 66;
    kickState = true;
    kickDirection = angleBallPlayer;
    xPosition= gameSituation.ballCurrentPose(1) + cosd(180 - angleBallGoal) * kickableAreaRadius;
    yPosition = gameSituation.ballCurrentPose(2) + sind(180 - angleBallGoal) * kickableAreaRadius;
    desiredPosition = [xPosition, yPosition, kickDirection];
    isdone = true;
  state Dribble
    en,du:
    angleBallGoal = atan2d(awayGoalPose(2) - gameSituation.ballCurrentPose(2), ...
    awayGoalPose(1) - gameSituation.ballCurrentPose(1));
    kickPower = 20;
    %%should be designed as the kickPower = kickPowerCofficent * 100
    %%kickPowerCofficieant should also be calculated by distance
    kickState = true;
    kickDirection = angleBallGoal;
    xPosition= gameSituation.ballCurrentPose(1) + cosd(180 - angleBallGoal) * kickableAreaRadius;
    yPosition = gameSituation.ballCurrentPose(2) + sind(180 - angleBallGoal) * kickableAreaRadius;
    desiredPosition = [xPosition, yPosition, kickDirection];
    isdone = true;
  state Intercept
    en,du:
    angleBallGoal = atan2d(awayGoalPose(2) - gameSituation.ballCurrentPose(2), ...
    awayGoalPose(1) - gameSituation.ballCurrentPose(1));
    kickPower = 50;
    kickState = true;
    kickDirection = angleBallGoal;
    xPosition= gameSituation.ballCurrentPose(1) + cosd(180 - angleBallGoal) * kickableAreaRadius;
    yPosition = gameSituation.ballCurrentPose(2) + sind(180 - angleBallGoal) * kickableAreaRadius;
    desiredPosition = [xPosition, yPosition, kickDirection];
    isdone = true;
  state Formation
    en,du:
    playerDefendPosition = homeDefendPositions(id, :);
    kickPower = 1;
    kickState = false;
    desiredPosition = playerDefendPosition;
    isdone = true;
  state Kick
    state MoveTo1
      en,du:
      isdone = false;
      robotCommand.robotDestinationPose = desiredPosition;
      distToBall = distTo(gameSituation.robotCurrentPose(id,1:2), ...
      gameSituation.ballCurrentPose(1:2));
    state KickTo
      en,du:
      robotCommand.kick = kickState;
      robotCommand.kickProperty = kickPower;
      isdone = true;
    MoveTo1 -> KickTo [order 1] : [distToBall <= kickableAreaRadius+5]
  MoveTo1 -> InitialState [order 2] : [after(2,sec)]
  KickTo -> InitialState : [after(5,sec)]
  (default) -> InitialState
  InitialState -> Attack [order 2] : [gameSituation.ballLastCommandBy(1) == 2]
  InitialState -> Defend [order 1] : [gameSituation.ballLastCommandBy(1) == 1]
  Attack -> Position [order 1] : [distToBall ~= min(teamDistToBall)]
  Defend -> Intercept [order 1] : [distToBall ~= max(teamDistToBall)]
  Defend -> Formation [order 2] : [distToBall == max(teamDistToBall)]
  Attack -> Pass [order 3] : [distToGoal1 ~= min(teamDistToGoal)&& distToBall == min(teamDistToBall)]
  Attack -> Dribble [order 4] : [distToBall == min(teamDistToBall) && distToGoal1 == min(teamDistToGoal) && distToGoal1 > shootDistThres]
  Attack -> Shoot [order 2] : [distToBall == min(teamDistToBall) && distToGoal1 == min(teamDistToGoal) && distToGoal1 < shootDistThres]
  Intercept -> MoveTo1 : [isdone]
  Formation -> MoveTo1 : [isdone]
  Pass -> MoveTo1 : [isdone]
  Dribble -> MoveTo1 : [isdone]
  Shoot -> MoveTo1 : [isdone]
  Position -> MoveTo1 : [isdone]
  data: robotPosition function_input; goalPosition function_input; dist function_output; awayGoalPose local =[0 0]; homeGoalPose local =[0 0]; id local =1; idx local; angleBallGoal local =0; desiredPosition local =[0 0 0]; distToOwnGoal local =0; kickDirection local =0; kickPower local =0; kickState local =false; minidx local; playerDefendPosition local =[0 0 0]; teamDistToGoal local =[0 0 0 0]; teamDistToOwnGoal local =[0 0 0 0]; minval local; isdone local boolean =false; playerAttackPosition local =[0 0 0]; shootDistThres local =0; gameSituation input Bus: gameSituation; kickableAreaRadius local =0; distToGoal1 local =0; angleBallPlayer local =0; robotCommand output Bus: robotCommand; distToBall local =0; teamDistToBall local =[0 0 0 0]; homeAttackPositions local =[0 0 0;0 0 0;0 0 0;0 0 0]; homeDefendPositions local =[0 0 0;0 0 0;0 0 0;0 0 0]; xPosition local; yPosition local
  function dist = distTo(robotPosition,goalPosition):
    | function dist = distTo(robotPosition,goalPosition)
    |     dist = norm(robotPosition - goalPosition);
    | end

== stateflow chart RoboSoccerSim/Robot Team Clients 2 (Away)/Subsystem/Away Player Strategy 2 ==
  state InitialState
    en,du:
    if gameSituation.kickConfirmation == true
    robotCommand.kick = false;
    end
    id = 2; % Team1(Home) Robot 1
    shootDistThres = 2500;
    kickableAreaRadius = 20;
    homeGoalPose = [5000, 0];
    awayGoalPose = [-5000, 0];
    homeAttackPositions = [[-2500, 0, 180]; [-1500, 2000, 180]; [-1500, -2000, 180]; [2000, 0, 180]];
    homeDefendPositions = [[1000, 0, 180]; [3000, 2000, 180]; [3000, -2000, 180]; [3500, 0, 180]];
  state ROBOT 1 [group]
    (Strategy for robot 1~3)
  state Attack
    en,du:
    %%calculate the distance to the goal
    teamDistToGoal = [0 0 0 0];
    for idx=1:1:4
    teamDistToGoal(idx) = distTo(gameSituation.robotCurrentPose(idx,1:2), awayGoalPose);
    end
    distToGoal1 = distTo(gameSituation.robotCurrentPose(id,1:2), awayGoalPose);
    %calculate the distance to the ball
    teamDistToBall = [0 0 0 0];
    for idx=1:1:4
    teamDistToBall(idx) = distTo(gameSituation.robotCurrentPose(idx,1:2), ...
    gameSituation.ballCurrentPose(1:2));
    end
    distToBall = distTo(gameSituation.robotCurrentPose(id,1:2), ...
    gameSituation.ballCurrentPose(1:2));
  state Defend
    en,du:
    %%calculate the distance to the home goal
    teamDistToOwnGoal = [0 0 0 0];
    for idx=1:1:4
    teamDistToOwnGoal(idx) = distTo(gameSituation.robotCurrentPose(idx,1:2), homeGoalPose);
    end
    distToOwnGoal = distTo(gameSituation.robotCurrentPose(id,1:2), homeGoalPose);
    for idx=1:1:4
    teamDistToBall(idx) = distTo(gameSituation.robotCurrentPose(idx,1:2), ...
    gameSituation.ballCurrentPose(1:2));
    end
    distToBall = distTo(gameSituation.robotCurrentPose(id,1:2), ...
    gameSituation.ballCurrentPose(1:2));
  state Position
    en,du:
    playerAttackPosition = homeAttackPositions(id, :);
    kickPower = 1;
    kickState = false;
    desiredPosition = playerAttackPosition;
    isdone = true;
  state Shoot
    en,du:
    angleBallGoal = atan2d(awayGoalPose(2) - gameSituation.ballCurrentPose(2), ...
    awayGoalPose(1) - gameSituation.ballCurrentPose(1));
    kickPower = 100;
    kickState = true;
    kickDirection = angleBallGoal;
    xPosition= gameSituation.ballCurrentPose(1) + cosd(180 - angleBallGoal) * kickableAreaRadius;
    yPosition = gameSituation.ballCurrentPose(2) + sind(180 - angleBallGoal) * kickableAreaRadius;
    desiredPosition = [xPosition, yPosition, kickDirection];
    isdone = true;
  state Pass
    en,du:
    [minval,minidx] = min(teamDistToGoal)
    angleBallPlayer = atan2d(gameSituation.robotCurrentPose(minidx, 2) - gameSituation.ballCurrentPose(2), ...
    gameSituation.robotCurrentPose(minidx, 1) - gameSituation.ballCurrentPose(1));
    kickPower = 66;
    kickState = true;
    kickDirection = angleBallPlayer;
    xPosition= gameSituation.ballCurrentPose(1) + cosd(180 - angleBallGoal) * kickableAreaRadius;
    yPosition = gameSituation.ballCurrentPose(2) + sind(180 - angleBallGoal) * kickableAreaRadius;
    desiredPosition = [xPosition, yPosition, kickDirection];
    isdone = true;
  state Dribble
    en,du:
    angleBallGoal = atan2d(awayGoalPose(2) - gameSituation.ballCurrentPose(2), ...
    awayGoalPose(1) - gameSituation.ballCurrentPose(1));
    kickPower = 10;
    %%should be designed as the kickPower = kickPowerCofficent * 100
    %%kickPowerCofficieant should also be calculated by distance
    kickState = true;
    kickDirection = angleBallGoal;
    xPosition= gameSituation.ballCurrentPose(1) + cosd(180 - angleBallGoal) * kickableAreaRadius;
    yPosition = gameSituation.ballCurrentPose(2) + sind(180 - angleBallGoal) * kickableAreaRadius;
    desiredPosition = [xPosition, yPosition, kickDirection];
    isdone = true;
  state Intercept
    en,du:
    angleBallGoal = atan2d(awayGoalPose(2) - gameSituation.ballCurrentPose(2), ...
    awayGoalPose(1) - gameSituation.ballCurrentPose(1));
    kickPower = 50;
    kickState = true;
    kickDirection = angleBallGoal;
    xPosition= gameSituation.ballCurrentPose(1) + cosd(180 - angleBallGoal) * kickableAreaRadius;
    yPosition = gameSituation.ballCurrentPose(2) + sind(180 - angleBallGoal) * kickableAreaRadius;
    desiredPosition = [xPosition, yPosition, kickDirection];
    isdone = true;
  state Formation
    en,du:
    playerDefendPosition = homeDefendPositions(id, :);
    kickPower = 1;
    kickState = false;
    desiredPosition = playerDefendPosition;
    isdone = true;
  state Kick
    state MoveTo1
      en,du:
      isdone = false;
      robotCommand.robotDestinationPose = desiredPosition;
      distToBall = distTo(gameSituation.robotCurrentPose(id,1:2), ...
      gameSituation.ballCurrentPose(1:2));
    state KickTo
      en,du:
      robotCommand.kick = kickState;
      robotCommand.kickProperty = kickPower;
      isdone = true;
    MoveTo1 -> KickTo [order 1] : [distToBall <= kickableAreaRadius+5]
  MoveTo1 -> InitialState [order 2] : [after(2,sec)]
  KickTo -> InitialState : [after(5,sec)]
  (default) -> InitialState
  InitialState -> Attack [order 2] : [gameSituation.ballLastCommandBy(1) == 2]
  InitialState -> Defend [order 1] : [gameSituation.ballLastCommandBy(1) == 1]
  Attack -> Position [order 1] : [distToBall ~= min(teamDistToBall)]
  Defend -> Intercept [order 1] : [distToBall ~= max(teamDistToBall)]
  Defend -> Formation [order 2] : [distToBall == max(teamDistToBall)]
  Attack -> Pass [order 3] : [distToGoal1 ~= min(teamDistToGoal)&& distToBall == min(teamDistToBall)]
  Attack -> Dribble [order 4] : [distToBall == min(teamDistToBall) && distToGoal1 == min(teamDistToGoal) && distToGoal1 > shootDistThres]
  Attack -> Shoot [order 2] : [distToBall == min(teamDistToBall) && distToGoal1 == min(teamDistToGoal) && distToGoal1 < shootDistThres]
  Intercept -> MoveTo1 : [isdone]
  Formation -> MoveTo1 : [isdone]
  Pass -> MoveTo1 : [isdone]
  Dribble -> MoveTo1 : [isdone]
  Shoot -> MoveTo1 : [isdone]
  Position -> MoveTo1 : [isdone]
  data: robotPosition function_input; goalPosition function_input; dist function_output; awayGoalPose local =[0 0]; homeGoalPose local =[0 0]; id local =1; idx local; angleBallGoal local =0; desiredPosition local =[0 0 0]; distToOwnGoal local =0; kickDirection local =0; kickPower local =0; kickState local =false; minidx local; playerDefendPosition local =[0 0 0]; teamDistToGoal local =[0 0 0 0]; teamDistToOwnGoal local =[0 0 0 0]; minval local; isdone local boolean =false; playerAttackPosition local =[0 0 0]; shootDistThres local =0; gameSituation input Bus: gameSituation; kickableAreaRadius local =0; distToGoal1 local =0; angleBallPlayer local =0; robotCommand output Bus: robotCommand; distToBall local =0; teamDistToBall local =[0 0 0 0]; homeAttackPositions local =[0 0 0;0 0 0;0 0 0;0 0 0]; homeDefendPositions local =[0 0 0;0 0 0;0 0 0;0 0 0]; xPosition local; yPosition local
  function dist = distTo(robotPosition,goalPosition):
    | function dist = distTo(robotPosition,goalPosition)
    |     dist = norm(robotPosition - goalPosition);
    | end
